simulink model "intel_motor_control_rl2freddie"  (Simulink 10.3)
settings: Solver=FixedStepDiscrete  StartTime=0.0  StopTime=0.7  FixedStep=62.5e-6 % 16 kHz  RelTol=1e-3  EnableMultiTasking=on
undefined symbols (not defined in the file or in its folder): DiscIntNeverNeededParam, I_max, Position_PI_Limit
libraries: simulink x9, dspsrcs4 x2, rllib x1
(part 2 of 2)

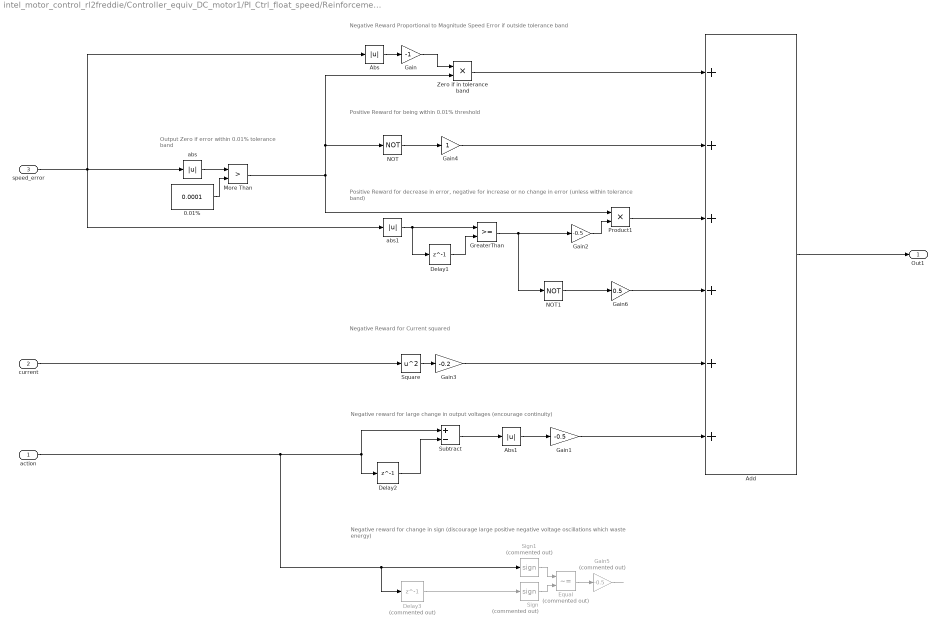
== system intel_motor_control_rl2freddie/Controller_equiv_DC_motor1/PI_Ctrl_float_speed/Reinforcement Learning1/Subsystem ==
  note: Negative Reward Proportional to Magnitude Speed Error
      | if outside tolerance band
  note: Output Zero if error within 0.01%
      | tolerance band
  note: Negative reward for large change in output voltages (encourage continuity)
  note: Positive Reward for decrease in error, negative for increase or no change
      | in error (unless within tolerance band)
  note: Positive Reward for being within 0.01% threshold
  note: Negative reward for change in sign
      | (discourage large positive negative voltage oscillations which waste energy)
  note: Negative Reward for Current squared
  action : Inport
  current : Inport  Port=2
  speed_error : Inport  Port=3
  0.01% : Constant  Value=0.0001
  Abs : Abs
  Abs1 : Abs
  Add : Sum  Inputs=++++++
  Delay1 : Delay  DelayLength=1
  Delay2 : Delay  DelayLength=1
  Delay3 : Delay  Commented=on  DelayLength=1
  Equal : RelationalOperator  Commented=on  Operator=~=  OutDataTypeStr=boolean  RndMeth=Simplest
  Gain : Gain  Gain=-1
  Gain1 : Gain  Gain=-0.5
  Gain2 : Gain  Gain=-0.5
  Gain3 : Gain  Gain=-0.2
  Gain4 : Gain
  Gain5 : Gain  Commented=on  Gain=-0.5
  Gain6 : Gain  Gain=0.5
  GreaterThan : RelationalOperator  OutDataTypeStr=boolean  RndMeth=Simplest
  More Than : RelationalOperator  Operator=>  OutDataTypeStr=boolean  RndMeth=Simplest
  NOT : Logic  Operator=NOT  IconShape=distinctive  AllPortsSameDT=off  OutDataTypeStr=boolean
  NOT1 : Logic  Operator=NOT  IconShape=distinctive  AllPortsSameDT=off  OutDataTypeStr=boolean
  Product1 : Product
  Sign : Signum  Commented=on
  Sign1 : Signum  Commented=on
  Square : Math  Operator=square  SaturateOnIntegerOverflow=on
  Subtract : Sum  Inputs=+-
  Zero if in tolerance band : Product
  abs : Abs
  abs1 : Abs
  Out1 : Outport
  wires:
  Gain5/1 -> ?
  Gain/1 -> Zero if in tolerance band/1
  Gain1/1 -> Add/6
  Gain6/1 -> Add/4
  abs1/1 -> GreaterThan/1, Delay1/1
  Gain3/1 -> Add/5
  speed_error/1 -> abs1/1, abs/1, Abs/1
  Sign1/1 -> Equal/1
  Product1/1 -> Add/3
  Delay1/1 -> GreaterThan/2
  More Than/1 -> Product1/1, Zero if in tolerance band/2, NOT/1
  Add/1 -> Out1/1
  Square/1 -> Gain3/1
  Gain2/1 -> Product1/2
  GreaterThan/1 -> Gain2/1, NOT1/1
  Delay2/1 -> Subtract/2
  current/1 -> Square/1
  Gain4/1 -> Add/2
  NOT/1 -> Gain4/1
  Subtract/1 -> Abs1/1
  Equal/1 -> Gain5/1
  Sign/1 -> Equal/2
  Zero if in tolerance band/1 -> Add/1
  Abs1/1 -> Gain1/1
  Abs/1 -> Gain/1
  Delay3/1 -> Sign/1
  action/1 -> Delay3/1, Sign1/1, Subtract/1, Delay2/1
  abs/1 -> More Than/1
  NOT1/1 -> Gain6/1
  0.01%/1 -> More Than/2

== system intel_motor_control_rl2freddie/Controller_3phase/Field_Oriented_Control/FOC_SimulinkFloat/FOC_Simulink_float/ClarkeTransform ==
  note: IAlpha =  Iu
      | IBeta = -1/sqrt(3)*(Iu + 2*Iw)
  Iu_A : Inport
  Iw_A : Inport  Port=2
  Constant : Constant  Value=-1/sqrt(3)
  Divide : Product  Inputs=**
  Gain : Gain
  Gain1 : Gain  Gain=2
  Sum : Sum  Inputs=++|
  IAlpha_A : Outport
  IBeta_A : Outport  Port=2
  wires:
  Divide/1 -> IBeta_A/1
  Iu_A/1 -> Gain/1
  Sum/1 -> Divide/1
  Iw_A/1 -> Gain1/1
  Gain1/1 -> Sum/2
  Gain/1 -> IAlpha_A/1, Sum/1  "IAlpha_A"
  Constant/1 -> Divide/2

== system intel_motor_control_rl2freddie/Controller_3phase/Field_Oriented_Control/FOC_SimulinkFloat/FOC_Simulink_float/InverseParkTransform ==
  note: Forward Park Transform: Iq = -IAlpha*Sin(Phi) + IBeta*Cos(Phi)
  note: Forward Park Transform: Id = IAlpha*Cos(Phi) + IBeta*Sin(Phi)
  note: Reverse Park Transform: VAlphaCmd_V = VdCmd_V*Cos(Phi) - VqCmd_V*Sin(Phi)
  note: Reverse Park Transform: VBetaCmd_V = VdCmd_V*Sin(Phi) + VqCmd_V*Cos(Phi)
  VdCmd_V : Inport
  VqCmd_V : Inport  Port=2
  SinPhi_ND : Inport  Port=3
  CosPhi_ND : Inport  Port=4
  CosPhi_ND1 : InportShadow  Port=4
  Product{,1..3} (4 alike) : Product
  SinPhi_ND1 : InportShadow  Port=3
  Sum : Sum  Inputs=|+-
  Sum1 : Sum  Inputs=|++
  VdCmd_V1 : InportShadow
  VqCmd_V1 : InportShadow  Port=2
  VAlphaCmd_V : Outport
  VBetaCmd_V : Outport  Port=2
  wires:
  Sum1/1 -> VBetaCmd_V/1
  Product3/1 -> Sum1/2
  Product2/1 -> Sum1/1
  CosPhi_ND1/1 -> Product3/2
  VqCmd_V1/1 -> Product3/1
  SinPhi_ND1/1 -> Product2/2
  VdCmd_V1/1 -> Product2/1
  Sum/1 -> VAlphaCmd_V/1
  Product1/1 -> Sum/2
  Product/1 -> Sum/1
  SinPhi_ND/1 -> Product1/2
  CosPhi_ND/1 -> Product/2
  VdCmd_V/1 -> Product/1
  VqCmd_V/1 -> Product1/1

== system intel_motor_control_rl2freddie/Controller_3phase/Field_Oriented_Control/FOC_SimulinkFloat/FOC_Simulink_float/ParkTransform ==
  note: Id = IAlpha*Cos(Phi) + IBeta*Sin(Phi)
  note: Iq = -IAlpha*Sin(Phi) + IBeta*Cos(Phi)
  IAlpha_A : Inport
  IBeta_A : Inport  Port=2
  SinPhi_ND : Inport  Port=3
  CosPhi_ND : Inport  Port=4
  CosPhi_ND1 : InportShadow  Port=4
  IAlpha_A1 : InportShadow
  IBeta_A1 : InportShadow  Port=2
  Product{,1..3} (4 alike) : Product
  SinPhi_ND1 : InportShadow  Port=3
  Sum : Sum  Inputs=|++
  Sum1 : Sum  Inputs=|-+
  Id_A : Outport
  Iq_A : Outport  Port=2
  wires:
  IBeta_A/1 -> Product1/1
  IAlpha_A/1 -> Product/1
  CosPhi_ND/1 -> Product/2
  SinPhi_ND/1 -> Product1/2
  Product/1 -> Sum/1
  Product1/1 -> Sum/2
  Sum/1 -> Id_A/1
  IAlpha_A1/1 -> Product2/1
  SinPhi_ND1/1 -> Product2/2
  IBeta_A1/1 -> Product3/1
  CosPhi_ND1/1 -> Product3/2
  Product2/1 -> Sum1/1
  Product3/1 -> Sum1/2
  Sum1/1 -> Iq_A/1

== system intel_motor_control_rl2freddie/Controller_3phase/Field_Oriented_Control/FOC_SimulinkFloat/FOC_Simulink_float/TwoPIControllers ==
  IdCmd_A_f : Inport
  IqCmd_A_f : Inport  Port=2
  IdFb_A_f : Inport  Port=3
  IqFb_A_f : Inport  Port=4
  FbErrorLimit_A_f : Inport  Port=5
  Kp_ND_f : Inport  Port=6
  Ki_NDperUpdate_f : Inport  Port=7
  IntegratorLimit_f : Inport  Port=8
  CmdLimit_f : Inport  Port=9
  DoReset_Bool : Inport  Port=10
  FbErrorLimit1_A_f : InportShadow  Port=5
  IntegratorLimit1 : InportShadow  Port=8
  Ki_NDperUpdate1 : InportShadow  Port=7
  Kp_ND1 : InportShadow  Port=6
  OutputLimit1 : InportShadow  Port=9
  PIController : Subsystem
  PIController1 : Subsystem
  ResetState_Bool1 : InportShadow  Port=10
  VdUnfilt_V : Outport
  VqUnfilt_V : Outport  Port=2
  wires:
  IdCmd_A_f/1 -> PIController/1(Cmd_f)
  PIController/1(NextCmd_f) -> VdUnfilt_V/1
  IdFb_A_f/1 -> PIController/2(Fb_f)
  PIController1/1(NextCmd_f) -> VqUnfilt_V/1
  ResetState_Bool1/1 -> PIController1/8(DoReset_Bool)
  OutputLimit1/1 -> PIController1/7(CmdLimit_f)
  IntegratorLimit1/1 -> PIController1/6(IntegratorLimit_f)
  Ki_NDperUpdate1/1 -> PIController1/5(Ki_NDperUpdate_f)
  Kp_ND1/1 -> PIController1/4(Kp_ND_f)
  FbErrorLimit1_A_f/1 -> PIController1/3(FbErrorLimit_f)
  IqFb_A_f/1 -> PIController1/2(Fb_f)
  IqCmd_A_f/1 -> PIController1/1(Cmd_f)
  DoReset_Bool/1 -> PIController/8(DoReset_Bool)
  CmdLimit_f/1 -> PIController/7(CmdLimit_f)
  IntegratorLimit_f/1 -> PIController/6(IntegratorLimit_f)
  Ki_NDperUpdate_f/1 -> PIController/5(Ki_NDperUpdate_f)
  Kp_ND_f/1 -> PIController/4(Kp_ND_f)
  FbErrorLimit_A_f/1 -> PIController/3(FbErrorLimit_f)

== system intel_motor_control_rl2freddie/Controller_equiv_DC_motor1/PI_Ctrl_float_speed/Reinforcement Learning1/Observations/limit_abs_value_of_integrator ==
  input : Inport
  abs_max : Inport  Port=2
  CmpLT : RelationalOperator  Operator=<  OutDataTypeStr=boolean  RndMeth=Nearest
  CmpLT1 : RelationalOperator  OutDataTypeStr=boolean  RndMeth=Nearest
  Switch : Switch  Criteria=u2 ~= 0  Threshold=Position_PI_Limit  ZeroCross=off
  Switch1 : Switch  Criteria=u2 ~= 0  Threshold=I_max  ZeroCross=off
  Unary Minus : UnaryMinus
  output : Outport
  wires:
  CmpLT1/1 -> Switch/2
  abs_max/1 -> Switch/1, CmpLT1/2, Unary Minus/1
  input/1 -> CmpLT1/1, Switch/3, CmpLT/1
  CmpLT/1 -> Switch1/2
  Switch/1 -> Switch1/3
  Switch1/1 -> output/1
  Unary Minus/1 -> Switch1/1, CmpLT/2

== system intel_motor_control_rl2freddie/Controller_equiv_DC_motor1/PI_Ctrl_float_speed/Reinforcement Learning1/Reward/limit_abs_value_of_integrator ==
  input : Inport
  abs_max : Inport  Port=2
  CmpLT : RelationalOperator  Operator=<  OutDataTypeStr=boolean  RndMeth=Nearest
  CmpLT1 : RelationalOperator  OutDataTypeStr=boolean  RndMeth=Nearest
  Switch : Switch  Criteria=u2 ~= 0  Threshold=Position_PI_Limit  ZeroCross=off
  Switch1 : Switch  Criteria=u2 ~= 0  Threshold=I_max  ZeroCross=off
  Unary Minus : UnaryMinus
  output : Outport
  wires:
  CmpLT1/1 -> Switch/2
  abs_max/1 -> Switch/1, CmpLT1/2, Unary Minus/1
  input/1 -> CmpLT1/1, Switch/3, CmpLT/1
  CmpLT/1 -> Switch1/2
  Switch/1 -> Switch1/3
  Switch1/1 -> output/1
  Unary Minus/1 -> Switch1/1, CmpLT/2

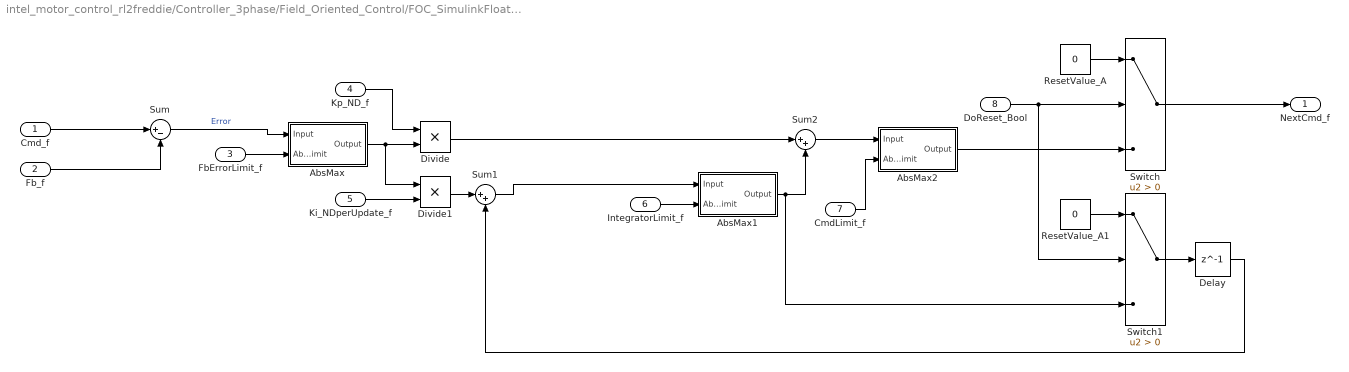
== system intel_motor_control_rl2freddie/Controller_3phase/Field_Oriented_Control/FOC_SimulinkFloat/FOC_Simulink_float/TwoPIControllers/PIController ==
  Cmd_f : Inport
  Fb_f : Inport  Port=2
  FbErrorLimit_f : Inport  Port=3
  Kp_ND_f : Inport  Port=4
  Ki_NDperUpdate_f : Inport  Port=5
  IntegratorLimit_f : Inport  Port=6
  CmdLimit_f : Inport  Port=7
  DoReset_Bool : Inport  Port=8
  AbsMax : Subsystem
  AbsMax1 : Subsystem
  AbsMax2 : Subsystem
  Delay : Delay  DelayLength=1  InitialCondition=0
  Divide : Product  Inputs=**
  Divide1 : Product  Inputs=**
  ResetValue_A : Constant  Value=0
  ResetValue_A1 : Constant  Value=0
  Sum : Sum  Inputs=|+-
  Sum1 : Sum  Inputs=|++
  Sum2 : Sum  Inputs=|++
  Switch : Switch  Criteria=u2 > Threshold
  Switch1 : Switch  Criteria=u2 > Threshold
  NextCmd_f : Outport
  wires:
  Fb_f/1 -> Sum/2
  Cmd_f/1 -> Sum/1
  Ki_NDperUpdate_f/1 -> Divide1/2
  Sum/1 -> AbsMax/1(Input)  "Error"
  Divide1/1 -> Sum1/1
  Kp_ND_f/1 -> Divide/1
  FbErrorLimit_f/1 -> AbsMax/2(AbsLimit)
  Sum1/1 -> AbsMax1/1(Input)
  Divide/1 -> Sum2/1
  AbsMax/1(Output) -> Divide1/1, Divide/2
  Delay/1 -> Sum1/2
  ResetValue_A1/1 -> Switch1/1
  CmdLimit_f/1 -> AbsMax2/2(AbsLimit)
  Sum2/1 -> AbsMax2/1(Input)
  AbsMax1/1(Output) -> Switch1/3, Sum2/2
  Switch/1 -> NextCmd_f/1
  ResetValue_A/1 -> Switch/1
  DoReset_Bool/1 -> Switch1/2, Switch/2
  AbsMax2/1(Output) -> Switch/3
  Switch1/1 -> Delay/1
  IntegratorLimit_f/1 -> AbsMax1/2(AbsLimit)

== system intel_motor_control_rl2freddie/Controller_3phase/Field_Oriented_Control/FOC_SimulinkFloat/FOC_Simulink_float/TwoPIControllers/PIController1 ==
  Cmd_f : Inport
  Fb_f : Inport  Port=2
  FbErrorLimit_f : Inport  Port=3
  Kp_ND_f : Inport  Port=4
  Ki_NDperUpdate_f : Inport  Port=5
  IntegratorLimit_f : Inport  Port=6
  CmdLimit_f : Inport  Port=7
  DoReset_Bool : Inport  Port=8
  AbsMax : Subsystem
  AbsMax1 : Subsystem
  AbsMax2 : Subsystem
  Delay : Delay  DelayLength=1  InitialCondition=0
  Divide : Product  Inputs=**
  Divide1 : Product  Inputs=**
  ResetValue_A : Constant  Value=0
  ResetValue_A1 : Constant  Value=0
  Sum : Sum  Inputs=|+-
  Sum1 : Sum  Inputs=|++
  Sum2 : Sum  Inputs=|++
  Switch : Switch  Criteria=u2 > Threshold
  Switch1 : Switch  Criteria=u2 > Threshold
  NextCmd_f : Outport
  wires:
  IntegratorLimit_f/1 -> AbsMax1/2(AbsLimit)
  Switch1/1 -> Delay/1
  AbsMax2/1(Output) -> Switch/3
  DoReset_Bool/1 -> Switch/2, Switch1/2
  ResetValue_A/1 -> Switch/1
  Switch/1 -> NextCmd_f/1
  AbsMax1/1(Output) -> Sum2/2, Switch1/3
  Sum2/1 -> AbsMax2/1(Input)
  CmdLimit_f/1 -> AbsMax2/2(AbsLimit)
  ResetValue_A1/1 -> Switch1/1
  Delay/1 -> Sum1/2
  AbsMax/1(Output) -> Divide/2, Divide1/1
  Divide/1 -> Sum2/1
  Sum1/1 -> AbsMax1/1(Input)
  FbErrorLimit_f/1 -> AbsMax/2(AbsLimit)
  Kp_ND_f/1 -> Divide/1
  Divide1/1 -> Sum1/1
  Sum/1 -> AbsMax/1(Input)  "Error"
  Ki_NDperUpdate_f/1 -> Divide1/2
  Cmd_f/1 -> Sum/1
  Fb_f/1 -> Sum/2

== system intel_motor_control_rl2freddie/Controller_3phase/Field_Oriented_Control/FOC_SimulinkFloat/FOC_Simulink_float/TwoPIControllers/PIController/AbsMax ==
  Input : Inport
  AbsLimit : Inport  Port=2
  Abs : Abs
  Divide : Product  Inputs=**
  Min : MinMax  Inputs=2
  Sign : Signum
  Output : Outport
  wires:
  AbsLimit/1 -> Min/2
  Abs/1 -> Min/1
  Divide/1 -> Output/1
  Min/1 -> Divide/1
  Sign/1 -> Divide/2
  Input/1 -> Sign/1, Abs/1

== system intel_motor_control_rl2freddie/Controller_3phase/Field_Oriented_Control/FOC_SimulinkFloat/FOC_Simulink_float/TwoPIControllers/PIController/AbsMax1 ==
  Input : Inport
  AbsLimit : Inport  Port=2
  Abs : Abs
  Divide : Product  Inputs=**
  Min : MinMax  Inputs=2
  Sign : Signum
  Output : Outport
  wires:
  Input/1 -> Abs/1, Sign/1
  Sign/1 -> Divide/2
  Min/1 -> Divide/1
  Divide/1 -> Output/1
  Abs/1 -> Min/1
  AbsLimit/1 -> Min/2

== system intel_motor_control_rl2freddie/Controller_3phase/Field_Oriented_Control/FOC_SimulinkFloat/FOC_Simulink_float/TwoPIControllers/PIController/AbsMax2 ==
  Input : Inport
  AbsLimit : Inport  Port=2
  Abs : Abs
  Divide : Product  Inputs=**
  Min : MinMax  Inputs=2
  Sign : Signum
  Output : Outport
  wires:
  AbsLimit/1 -> Min/2
  Abs/1 -> Min/1
  Divide/1 -> Output/1
  Min/1 -> Divide/1
  Sign/1 -> Divide/2
  Input/1 -> Sign/1, Abs/1

== system intel_motor_control_rl2freddie/Controller_3phase/Field_Oriented_Control/FOC_SimulinkFloat/FOC_Simulink_float/TwoPIControllers/PIController1/AbsMax ==
  Input : Inport
  AbsLimit : Inport  Port=2
  Abs : Abs
  Divide : Product  Inputs=**
  Min : MinMax  Inputs=2
  Sign : Signum
  Output : Outport
  wires:
  Input/1 -> Abs/1, Sign/1
  Sign/1 -> Divide/2
  Min/1 -> Divide/1
  Divide/1 -> Output/1
  Abs/1 -> Min/1
  AbsLimit/1 -> Min/2

== system intel_motor_control_rl2freddie/Controller_3phase/Field_Oriented_Control/FOC_SimulinkFloat/FOC_Simulink_float/TwoPIControllers/PIController1/AbsMax1 ==
  Input : Inport
  AbsLimit : Inport  Port=2
  Abs : Abs
  Divide : Product  Inputs=**
  Min : MinMax  Inputs=2
  Sign : Signum
  Output : Outport
  wires:
  AbsLimit/1 -> Min/2
  Abs/1 -> Min/1
  Divide/1 -> Output/1
  Min/1 -> Divide/1
  Sign/1 -> Divide/2
  Input/1 -> Sign/1, Abs/1

== system intel_motor_control_rl2freddie/Controller_3phase/Field_Oriented_Control/FOC_SimulinkFloat/FOC_Simulink_float/TwoPIControllers/PIController1/AbsMax2 ==
  Input : Inport
  AbsLimit : Inport  Port=2
  Abs : Abs
  Divide : Product  Inputs=**
  Min : MinMax  Inputs=2
  Sign : Signum
  Output : Outport
  wires:
  Input/1 -> Abs/1, Sign/1
  Sign/1 -> Divide/2
  Min/1 -> Divide/1
  Divide/1 -> Output/1
  Abs/1 -> Min/1
  AbsLimit/1 -> Min/2
